simulink model "patient_diabete_covid"  (R2019b)
settings: Solver=FixedStepDiscrete  StartTime=0.0  StopTime=10.0  FixedStep=0.1  RelTol=1e-3  EnableMultiTasking=on
settings Model: EnablePacing=on  PacingRate=1.400000  Creator=Paul Guilot  LastModifiedBy=Paul Guilot
settings SolverCC: AutoInsertRateTranBlk=on
settings DataIOCC: LimitDataPoints=on
settings OptimizationCC: LifeSpan=inf
settings DebuggingCC: AllowSymbolicDim=off  SFUnexpectedBacktrackingDiag=warning  SFNoUnconditionalDefaultTransitionDiag=warning  SFExecutionAtInitializationDiag=none  ArithmeticOperatorsInVariantConditions=warning
settings SFSimCC: SimUseLocalCustomCode=off  CustomCodeUndefinedFunction=UseInterfaceOnly
settings RTWCC: RTWUseLocalCustomCode=off
settings CodeAppCC: StateflowObjectComments=on
settings GRTTargetCC: TargetLangStandard=C89/C90 (ANSI)  GeneratePreprocessorConditionals=Disable all
settings ConfigComp: CovMetricSettings=dw  CovHtmlReporting=on  CovSaveCumulativeToWorkspaceVar=on  CovSaveSingleToWorkspaceVar=on  CovShowResultsExplorer=off  CovExternalEMLEnable=off  CovSFcnEnable=off

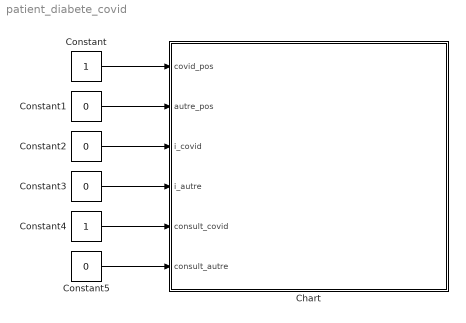
== system patient_diabete_covid ==
  Chart : Stateflow chart  TreatAsAtomicUnit=on
  Constant : Constant
  Constant{1..3,5} (4 alike) : Constant  Value=0
  Constant4 : Constant
  wires:
  Constant/1 -> Chart/1(covid_pos)
  Constant2/1 -> Chart/3(i_covid)
  Constant1/1 -> Chart/2(autre_pos)
  Constant3/1 -> Chart/4(i_autre)
  Constant4/1 -> Chart/5(consult_covid)
  Constant5/1 -> Chart/6(consult_autre)

== stateflow chart patient_diabete_covid/Chart ==
  state Consultation
    state Medecin_traitant
      if consult_covid == 1
      inscrit_covid = 1
      end
    state Medecin_specialiste_autre
      test_autre = 1
      inscrit_autre = 1
    (default) -> Medecin_traitant
    Medecin_traitant -> Consultation.Medecin_specialiste_autre : [autre_pos == 1]
  state Initialisation
    fin = 0
    inscrit_autre = i_autre
    inscrit_covid = i_covid
    if inscrit_autre == 1
    test_autre = 1
    else
    test_autre = 0
    end
    if inscrit_covid == 1
    test_covid = 1
    else
    test_covid = 0
    end
  state Plateforme
    state Suivi [parallel]
      settings: executionOrder=1
      state Suivi_Covid
      state Suivi_autre_et_Covid
      state Suivi_autre
      (default) -> Suivi_Covid [order 1] : [inscrit_covid == 1 & inscrit_autre == 0]
      Suivi_Covid -> Suivi_autre_et_Covid : [inscrit_autre == 1]
      Suivi_autre_et_Covid -> Suivi_Covid [order 1] : [inscrit_autre == 0]
      (default) -> Suivi_autre_et_Covid [order 2] : [inscrit_autre == 1 & inscrit_covid == 1]
      Suivi_autre_et_Covid -> Suivi_autre [order 2] : [inscrit_covid == 0]
      Suivi_autre -> Suivi_autre_et_Covid : [inscrit_covid == 1]
      (default) -> Suivi_autre [order 3] : [inscrit_covid == 0 & inscrit_autre == 1]
    state Choix [parallel]
      settings: executionOrder=2
      state Covid_et_Autre
        state Test_Covid
          if covid_pos == 1
          test_covid = 1
          end
        state Deja_teste
        (default) -> Plateforme.Choix.Covid_et_Autre.Test_Covid [order 1] : [consult_covid == 1 & test_covid == 0]
        Plateforme.Choix.Covid_et_Autre.Test_Covid -> Plateforme.Choix.Covid_et_Autre.Deja_teste : after(d, sec)
        (default) -> Plateforme.Choix.Covid_et_Autre.Deja_teste [order 2]
      state Covid
        state Test_Covid1
          if covid_pos == 1
          test_covid = 1
          end
        state Deja_teste
        (default) -> Test_Covid1 [order 1] : [consult_covid == 1 & test_covid == 0]
        Test_Covid1 -> Plateforme.Choix.Covid.Deja_teste : after(d, sec)
        (default) -> Plateforme.Choix.Covid.Deja_teste [order 2]
      state Autre
      state Test_Covid
        test_covid = 1
      state Medecin_generaliste
      state Medecin_specialiste_autre
        test_autre = 1
      state Guerison
        inscrit_covid = 0
        test_covid = 0
      (default) -> Covid_et_Autre [order 3] : [inscrit_covid == 1 & inscrit_autre == 1]
      (default) -> Covid [order 1] : [inscrit_covid == 1 & inscrit_autre == 0]
      (default) -> Autre [order 2] : [inscrit_autre == 1 & inscrit_covid == 0]
      Covid_et_Autre -> Autre [order 1] : after(guerison, sec) {test_covid = 0 ; inscrit_covid = 0 ; fin = 1}
      Autre -> Autre [order 1] : [fin == 1]
      Covid_et_Autre -> Autre [order 2] : after(d, sec) [test_covid == 0] {fin = 1}
      Autre -> Medecin_generaliste [order 2] : [consult_covid == 1]
      Autre -> Plateforme.Choix.Test_Covid [order 3] : [covid_pos == 1]
      Covid -> Guerison [order 3] : after(d, sec) [test_covid == 0]
      Covid -> Guerison [order 2] : after(guerison, sec)
      Covid -> Medecin_generaliste [order 1] : [consult_autre == 1]
      Plateforme.Choix.Test_Covid -> Covid_et_Autre : after(d, sec) {inscrit_covid = 1}
      Plateforme.Choix.Medecin_specialiste_autre -> Covid_et_Autre : {inscrit_autre =1}
      Medecin_generaliste -> Covid_et_Autre [order 1] : [inscrit_covid == 0] {inscrit_covid =1}
      Medecin_generaliste -> Plateforme.Choix.Medecin_specialiste_autre [order 2] : [autre_pos == 1]
  state Absent_de_la_plateforme
  state Initialisation1
    fin = 0
    test_covid = 0
    test_autre = 0
    inscrit_autre = i_autre
    inscrit_covid = i_covid
  state Test_Covid
    during :
    if covid_pos == 1
    test_covid = 1
    else
    test_covid = 0
    end
  (default) -> Initialisation [order 1] : [or(i_autre == 1, i_covid == 1)]
  Consultation -> Absent_de_la_plateforme [order 2] : [autre_pos == 0 & covid_pos == 0] {fin = 1}
  Absent_de_la_plateforme -> Consultation [order 2] : [or(consult_covid == 1, consult_autre == 1)]
  Initialisation -> Plateforme
  Consultation -> Plateforme [order 1] : [or([inscrit_autre == 1], [inscrit_covid == 1 & autre_pos == 0])]
  Absent_de_la_plateforme -> Absent_de_la_plateforme [order 1] : [fin == 1]
  Initialisation1 -> Absent_de_la_plateforme
  (default) -> Initialisation1 [order 2] : [i_autre == 0 & i_covid == 0]
  Plateforme -> Absent_de_la_plateforme : [inscrit_covid == 0 & inscrit_autre == 0]{fin = 1}
  Test_Covid -> Absent_de_la_plateforme [order 2] : after(d, sec) [test_covid == 0] {fin = 1}
  Absent_de_la_plateforme -> Test_Covid [order 3]
  Test_Covid -> Plateforme [order 1] : after(d, sec) [test_covid == 1] {inscrit_covid = 1}
  data: covid_pos input; autre_pos input; test_covid local; d constant double =2; guerison constant double =5; inscrit_covid local; i_covid input; i_autre input; consult_covid input; fin local; test_autre local; inscrit_autre local; consult_autre input
